simulink model "linear_vs_discrete"  (R2019b)
settings: Solver=VariableStepAuto  StartTime=0.0  StopTime=100  RelTol=1e-3
values from neighbouring files (symbols this model uses):
  c1 = -(T1+T2)/(T1*T2)    (= -0.576923076923)    [setup.m]
  c2 = -1/(T1*T2)    (= -0.0384615384615)    [setup.m]
  c4 = K/(T1*T2)    (= 0.230769230769)    [setup.m]
  T = 0.5    [setup.m]
  u_ = 1    [setup.m]
settings Model: Creator=marcel  LastModifiedBy=marcel

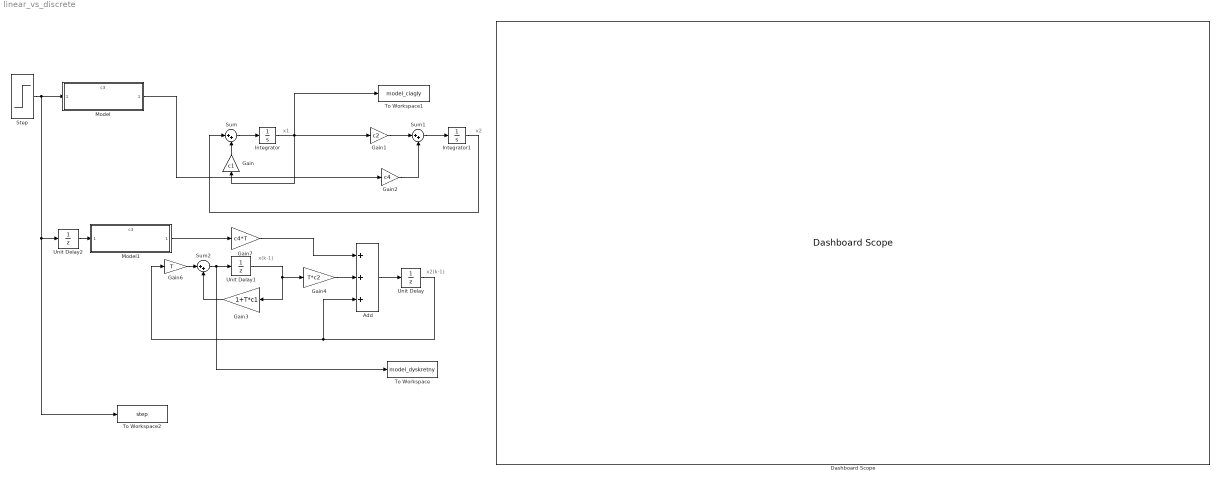
== system linear_vs_discrete ==
  note: x2(k-1)
  note: x(k-1)
  note: x2
  note: x1
  Add : Sum  Inputs=+++
  Dashboard Scope : DashboardScope
  Gain : Gain  Gain=c1
  Gain1 : Gain  Gain=c2
  Gain2 : Gain  Gain=c4
  Gain3 : Gain  Gain=1+T*c1
  Gain4 : Gain  Gain=T*c2
  Gain6 : Gain  Gain=T
  Gain7 : Gain  Gain=c4*T
  Integrator : Integrator
  Integrator1 : Integrator
  Model : ModelReference  ModelNameDialog=c3.slx  SimulationMode=Normal  ModelReferenceVersion=1.1
  Model1 : ModelReference  ModelNameDialog=c3.slx  SimulationMode=Normal  ModelReferenceVersion=1.1
  Step : Step  After=u_  SampleTime=T
  Sum : Sum  Inputs=|++
  Sum1 : Sum  Inputs=|++
  Sum2 : Sum  Inputs=|++
  To Workspace : ToWorkspace  VariableName=model_dyskretny  SaveFormat=Timeseries  SampleTime=-1
  To Workspace1 : ToWorkspace  VariableName=model_ciagly  SaveFormat=Timeseries  SampleTime=-1
  To Workspace2 : ToWorkspace  VariableName=step  SaveFormat=Timeseries  SampleTime=-1
  Unit Delay : UnitDelay  SampleTime=-1  HasFrameUpgradeWarning=on
  Unit Delay1 : UnitDelay  SampleTime=-1  HasFrameUpgradeWarning=on
  Unit Delay2 : UnitDelay  SampleTime=-1  HasFrameUpgradeWarning=on
  wires:
  Integrator/1 -> To Workspace1/1, Gain1/1, Gain/1
  Gain/1 -> Sum/2
  Sum/1 -> Integrator/1
  Gain1/1 -> Sum1/1
  Sum1/1 -> Integrator1/1
  Model/1 -> Gain2/1
  Integrator1/1 -> Sum/1
  Gain2/1 -> Sum1/2
  Unit Delay1/1 -> Gain4/1, Gain3/1
  Gain3/1 -> Sum2/2
  Sum2/1 -> Unit Delay1/1, To Workspace/1
  Add/1 -> Unit Delay/1
  Unit Delay/1 -> Gain6/1, Add/3
  Gain6/1 -> Sum2/1
  Unit Delay2/1 -> Model1/1
  Model1/1 -> Gain7/1
  Gain4/1 -> Add/2
  Gain7/1 -> Add/1
  Step/1 -> Unit Delay2/1, To Workspace2/1, Model/1
  ? -> ?
  ? -> ?
